simulink model "simosys"  (Simulink 2.20)
settings: Solver=ode45  StartTime=0.0  StopTime=20  MaxStep=10  RelTol=1e-3  AbsTol=1e-6
settings Model: ExternalInput=[]  SaveTime=off  SaveOutput=off  InitialState=[]  ConsistencyChecking=off  RTWPlaceOutputsASAP=off  RTWLocalBlockOutputs=on

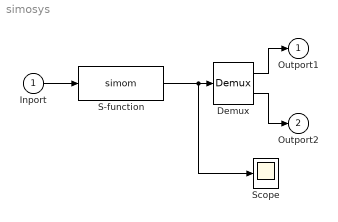
== system simosys ==
  Inport : Inport  Port=1  PortWidth=-1  SampleTime=-1
  Demux : Demux  Outputs=2
  S-function : S-Function  FunctionName=simom  PortCounts=[]  SFunctionModules=''
  Scope : Scope
      settings: TickLabels=on  TimeRange=20  YMin=-2  YMax=6  SaveToWorkspace=off  SaveName=ScopeData
  Outport1 : Outport  Port=1  InitialOutput=0
  Outport2 : Outport  Port=2  InitialOutput=0
  wires:
  Demux/2 -> Outport2/1
  Demux/1 -> Outport1/1
  S-function/1 -> Demux/1, Scope/1
  Inport/1 -> S-function/1
